simulink model "components_threewinding_transformer"  (R2016a)
settings: Solver=ode45  StartTime=0.0  StopTime=10.0  RelTol=1e-3
libraries: powerlib x10, powerlib_meascontrol x2, simulink x1
settings Model: Creator=obulreddy  LastModifiedBy=Sayan
settings DataIOCC: LimitDataPoints=on  SaveFormat=Array
settings HardwareCC: ProdBitPerPointer=32  ProdLargestAtomicFloat=None  ProdIntDivRoundTo=Undefined  ProdEndianess=Unspecified  ProdWordSize=32  ProdHWDeviceType=32-bit Generic
settings ModelReferenceCC: PropagateSignalLabelsOutOfModel=off
settings SimscapeCC: SimscapeNormalizeSystem=off

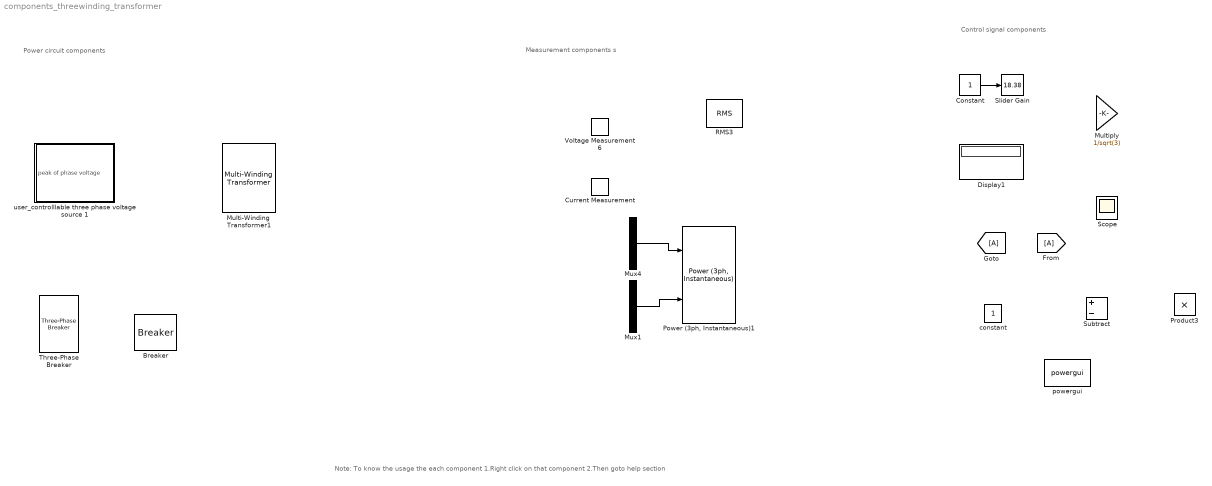
== system components_threewinding_transformer ==
  note: Note:
      | To know the usage the each component
      | 1.Right click on that component
      | 2.Then goto help section
  note: Measurement components s
  note: Control signal components
  note: Power circuit components
  Breaker : powerlib/Elements/Breaker  InitialState=0  SwitchingTimes="[1/60  5/60]"  External=on  BreakerResistance=0.01  SnubberResistance=1e6  SnubberCapacitance=inf  Measurements=None  MoreParameters=on  NoBreakLoop=off
  "Constant " : Constant
  Current Measurement : powerlib/Measurements/Current Measurement  PhasorSimulation=off  OutputType=Complex  PSBequivalent=0
  Display1 : Display
  Multi-Winding Transformer1 : powerlib/Elements/Multi-Winding Transformer  LeftWindings=1  RightWindings=2  TappedWindings=no taps  NumberOfTaps=2  SetSaturation=off  Hysteresis=off  DataFile='hysteresis.mat'  Measurements=None  UNITS=SI  NominalPower=[2e3 50]  NominalVoltages="[ 133  66  115 ]"  WindingResistances=[0.040222 0.00689 0.029063]  WindingInductances=[0.00052306 0.00009866 0.00038096]  Rm=392.23  Lm=1.0076  Saturation=[0 0;0.051039 0.71845;21.266 0.91004]  BreakLoop=off  DiscreteSolver=Trapezoidal iterative  DataType=on  InitialFlux=0  TransfoNumber=1
  Multiply : Gain  Gain=1/sqrt(3)
  Mux1 : Mux  Inputs=3
  Mux4 : Mux  Inputs=3
  "Power (3ph, Instantaneous)1" : powerlib_meascontrol/Measurements/Power (3ph, Instantaneous)
  Product3 : Product
  RMS3 : powerlib_meascontrol/Measurements/RMS  TrueRMS=on  Freq=50  RMSInit=0  Ts=0
  Scope : Scope
  Slider Gain : simulink/Math Operations/Slider Gain  gain=18.38  low=0  high=162
  Subtract : Sum  Inputs=+-
  Three-Phase Breaker : powerlib/Elements/Three-Phase Breaker  InitialState=open  SwitchA=on  SwitchB=on  SwitchC=on  SwitchTimes="[1/60  5/60]"  External=on  BreakerResistance=0.001  SnubberResistance=1e6  SnubberCapacitance=inf  Measurements=None
  Voltage Measurement6 : powerlib/Measurements/Voltage Measurement  PhasorSimulation=off  OutputType=Complex  PSBequivalent=0
  "constant " : Constant  OutDataTypeStr=Inherit: Inherit via back propagation
  powergui : powerlib/powergui  Priority=1  SimulationMode=Continuous  SampleTime=50e-6  frequency=60  Iterations=50  frequencyindice=50  Pbase=100e6  ErrMax=1e-4  UnitsV=kV  UnitsW=MW  buscounter=0  FunctionMessages=off  echomessages=off  EnableUseOfTLC=off  CurrentSourceSwitches=off  DisableSnubberDevices=off  DisableRonSwitches=off  DisableVfSwitches=off  DisplayEquations=off  AutomaticDiscreteSolvers=off  SolverType=Tustin/Backward Euler (TBE)  Interpol=off  ExternalGateDelay=off  methode=off  Ts=100  x0status=blocks  SPID=on  SwTol=0  HookPort=off  NonlinearTolerance=1e-4  nMaxIteration=100  ContinueOnMaxIteration=off  RestoreLinks=warning  ResistiveCurrentMeasurement=off  Frange=[0:2:500]  Ylog=off  Xlog=on  ShowGrid=off  save=off  variable=ZData  structure=0  ZoomFFT=off  StartTime=0.0  cycles=1  DisplayStyle=1  fundamental=60  FreqAxis=off  MaxFrequency=1000  frequencyindicesteady=1  RmsSteady=1  display=off
  user_controlllable three phase voltage source 1 : Subsystem
  wires:
  "Constant "/1 -> Slider Gain/1
  Mux4/1 -> "Power (3ph, Instantaneous)1"/1
  Mux1/1 -> "Power (3ph, Instantaneous)1"/2

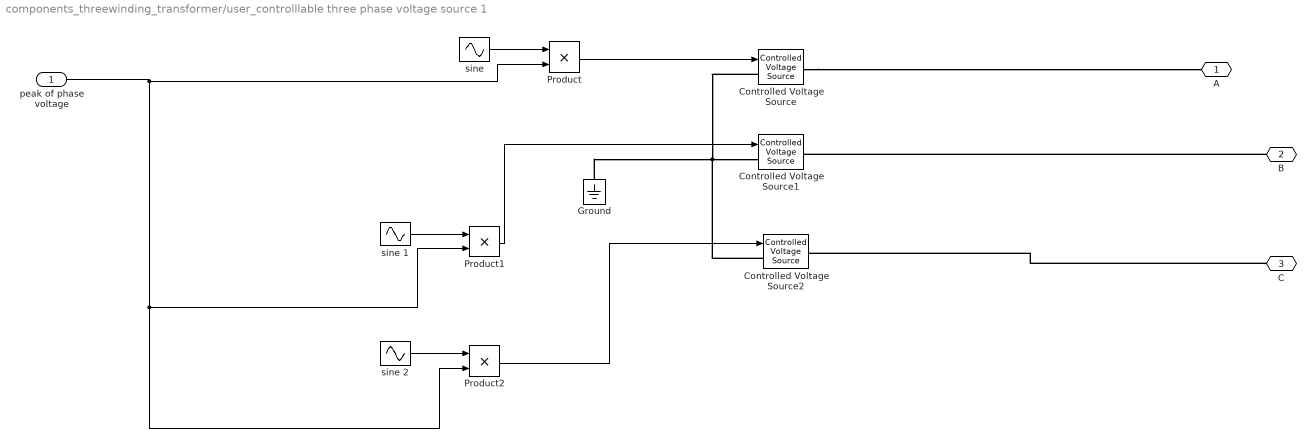
== system components_threewinding_transformer/user_controlllable three phase voltage source 1 ==
  peak of phase voltage : Inport
  Controlled Voltage Source : powerlib/Electrical Sources/Controlled Voltage Source  Initialize=off  Source_Type=DC  Amplitude=0  Phase=0  Frequency=50  Measurements=None
  Controlled Voltage Source1 : powerlib/Electrical Sources/Controlled Voltage Source  Initialize=off  Source_Type=DC  Amplitude=0  Phase=-120  Frequency=50  Measurements=None
  Controlled Voltage Source2 : powerlib/Electrical Sources/Controlled Voltage Source  Initialize=off  Source_Type=DC  Amplitude=0  Phase=120  Frequency=50  Measurements=None
  Ground : powerlib/Elements/Ground  LConnTagsString=a
  Product : Product
  Product1 : Product
  Product2 : Product
  "sine " : Sin  Frequency=2*pi*50  SampleTime=0
  sine 1 : Sin  Frequency=2*pi*50  Phase=-2*pi/3  SampleTime=0
  sine 2 : Sin  Frequency=2*pi*50  Phase=+2*pi/3  SampleTime=0
  A : PMIOPort  Side=Right
  B : PMIOPort  Port=2  Side=Right
  C : PMIOPort  Port=3  Side=Right
  wires:
  Product/1 -> Controlled Voltage Source/1
  sine 2/1 -> Product2/1
  Product2/1 -> Controlled Voltage Source2/1
  "sine "/1 -> Product/1
  sine 1/1 -> Product1/1
  Product1/1 -> Controlled Voltage Source1/1
  peak of phase voltage/1 -> Product2/2, Product1/2, Product/2
  connections:
  Controlled Voltage Source/RConn1 -- A/RConn1
  Controlled Voltage Source/LConn1 -- Controlled Voltage Source2/LConn1 -- Ground/LConn1 -- Controlled Voltage Source1/LConn1
  B/RConn1 -- Controlled Voltage Source1/RConn1
  C/RConn1 -- Controlled Voltage Source2/RConn1
